simulink model "SAPF_pq_theory_Without_PI_Controller"  (R2023a)
settings: Solver=VariableStepAuto  StartTime=0.0  StopTime=2  RelTol=1e-3
libraries: spsThreePhaseVIMeasurementLib x3, spsSeriesRLCBranchLib x2, spsUniversalBridgeLib x2, dspfdesign x1, spsThreePhaseSeriesRLCBranchLib x1, spsThreePhaseSourceLib x1, spsVoltageMeasurementLib x1, sps_lib x1
settings Model: Creator=Nitiz Khanal  LastModifiedBy=Nitiz Khanal
settings DataIOCC: ReturnWorkspaceOutputs=off

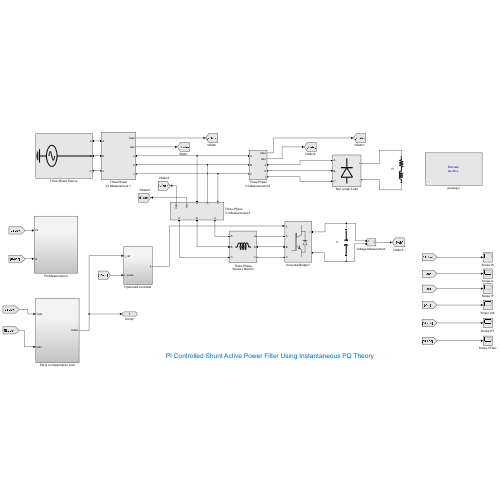
[thumbnail: Simulink's stored preview of the top-level diagram]
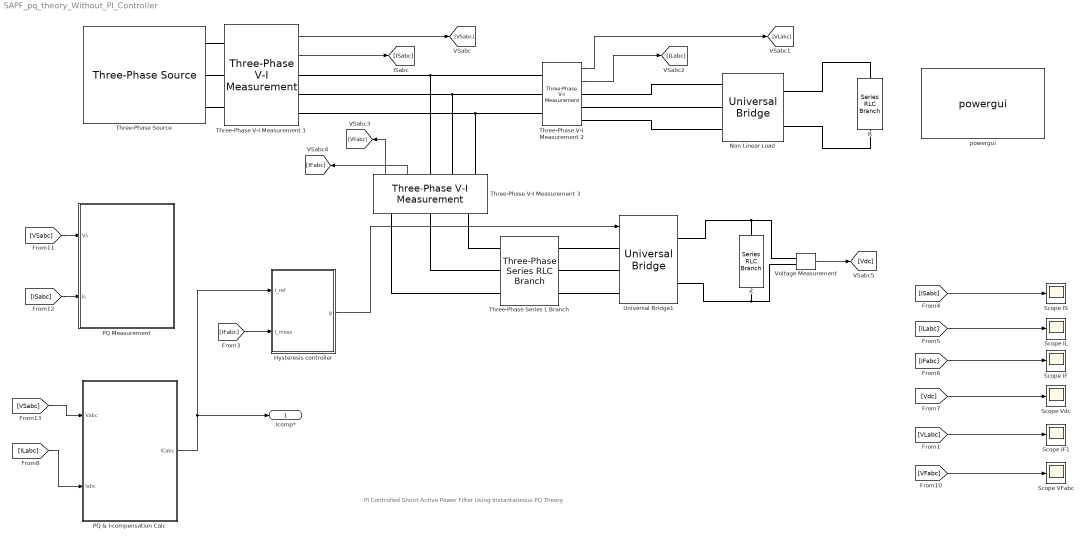
== system SAPF_pq_theory_Without_PI_Controller ==
  note: PI Controlled Shunt Active Power Filter Using Instantaneous PQ Theory
  C : spsSeriesRLCBranchLib/Series RLC Branch  LConnTagsString=__new0  RConnTagsString=__new0  BranchType=C  Resistance=1  Inductance=1e-3  SetiL0=off  InitialCurrent=0  Capacitance=1500e-6  Setx0=on  InitialVoltage=500  Measurements=None
  Hysteresis controller : Subsystem
  Non Linear Load : spsUniversalBridgeLib/Universal Bridge  Arms=3  SnubberResistance=1e5  SnubberCapacitance=inf  Device=Diodes  Ron=1e-3  Lon=0  ForwardVoltages="[  0  0  ]"  ForwardVoltage=0  GTOparameters=[ 10e-6 , 20e-6 ]  IGBTparameters=[ 1e-6 , 2e-6 ]  Measurements=None  Measurements_2=None  converterType=Rectifier
  PQ & I-compensation Calc : Subsystem
  PQ Measurement : Subsystem
  R : spsSeriesRLCBranchLib/Series RLC Branch  LConnTagsString=__new0  RConnTagsString=__new0  BranchType=RL  Resistance=30  Inductance=100e-3  SetiL0=off  InitialCurrent=0  Capacitance=1e-6  Setx0=off  InitialVoltage=0  Measurements=None
  Scope IF : Scope
  Scope IF1 : Scope
  Scope IL : Scope
  Scope IS : Scope
  Scope VFabc : Scope
  Scope Vdc : Scope
  Three-Phase Series L Branch : spsThreePhaseSeriesRLCBranchLib/Three-Phase Series RLC Branch  LConnTagsString=A|B|C  RConnTagsString=A|B|C  BranchType=L  Resistance=1  Inductance=2e-3  Capacitance=1e-6  Measurements=None
  "Three-Phase V-I Measurement 1 " : spsThreePhaseVIMeasurementLib/Three-Phase V-I Measurement  VoltageMeasurement=phase-to-ground  SetLabelV=off  LabelV=Vabc  Vpu=off  VpuLL=off  CurrentMeasurement=yes  SetLabelI=off  LabelI=Iabc  Ipu=off  Pbase=100e6  Vbase=500e3  OutputType=Complex  PhasorSimulation=off  PSBequivalent=0
  "Three-Phase V-I Measurement 2 " : spsThreePhaseVIMeasurementLib/Three-Phase V-I Measurement  VoltageMeasurement=phase-to-ground  SetLabelV=off  LabelV=Vabc  Vpu=off  VpuLL=off  CurrentMeasurement=yes  SetLabelI=off  LabelI=Iabc  Ipu=off  Pbase=100e6  Vbase=500e3  OutputType=Complex  PhasorSimulation=off  PSBequivalent=0
  Three-Phase V-I Measurement 3 : spsThreePhaseVIMeasurementLib/Three-Phase V-I Measurement  VoltageMeasurement=phase-to-ground  SetLabelV=off  LabelV=Vabc  Vpu=off  VpuLL=off  CurrentMeasurement=yes  SetLabelI=off  LabelI=Iabc  Ipu=off  Pbase=100e6  Vbase=500e3  OutputType=Complex  PhasorSimulation=off  PSBequivalent=0
  "Three-Phase Source " : spsThreePhaseSourceLib/Three-Phase Source  InternalConnection=Yg  VoltagePhases=off  Voltage=220  PhaseAngle=0  Voltage_phases=[25e3 25e3 25e3]/sqrt(3)  PhaseAngles_phases=[0 -120 +120]  Frequency=50  NonIdealSource=off  SpecifyImpedance=off  Resistance=0.8929  Inductance=16.58e-3  ShortCircuitLevel=100e6  BaseVoltage=25e3  XRratio=7  BusType=swing  Pref=10e3  Qref=0  Prefabc=[10e3, 10e3, 10e3]  Qrefabc=[0, 0, 0]  Qmin=-inf  Qmax=inf
  "Universal Bridge1 " : spsUniversalBridgeLib/Universal Bridge  Arms=3  SnubberResistance=1e5  SnubberCapacitance=inf  Device=IGBT / Diodes  Ron=1e-3  Lon=0  ForwardVoltages="[  0  0  ]"  ForwardVoltage=0  GTOparameters=[ 10e-6 , 20e-6 ]  IGBTparameters=[ 1e-6 , 2e-6 ]  Measurements=None  Measurements_2=None  converterType=Rectifier
  "Voltage Measurement " : spsVoltageMeasurementLib/Voltage Measurement  PhasorSimulation=off  OutputType=Complex  PSBequivalent=0
  powergui : sps_lib/powergui  Priority=1  SimulationMode=Discrete  SampleTime=2e-6  frequency=60  Iterations=50  frequencyindice=50  Pbase=100e6  ErrMax=1e-4  UnitsV=kV  UnitsW=MW  buscounter=0  FunctionMessages=off  echomessages=off  EnableUseOfTLC=off  CurrentSourceSwitches=off  DisableSnubberDevices=off  DisableRonSwitches=off  DisableVfSwitches=off  DisplayEquations=off  AutomaticDiscreteSolvers=off  SolverType=Tustin/Backward Euler (TBE)  Interpol=off  ExternalGateDelay=off  methode=off  Ts=100  x0status=blocks  SPID=on  SwTol=0  HookPort=off  NonlinearTolerance=1e-4  nMaxIteration=100  ContinueOnMaxIteration=off  RestoreLinks=warning  ResistiveCurrentMeasurement=off  Frange=[0:2:500]  Ylog=off  Xlog=on  ShowGrid=off  save=off  variable=ZData  structure=0  ZoomFFT=off  StartTime=0.0  cycles=1  DisplayStyle=1  fundamental=60  FreqAxis=off  MaxFrequency=1000  frequencyindicesteady=1  RmsSteady=1  display=off
  Icomp* : Outport
  wires:
  "Three-Phase V-I Measurement 1 "/1 -> [VSabc]
  "Three-Phase V-I Measurement 1 "/2 -> [ISabc]
  "Three-Phase V-I Measurement 2 "/1 -> [VLabc]
  "Three-Phase V-I Measurement 2 "/2 -> [ILabc]
  Three-Phase V-I Measurement 3/1 -> [VFabc]
  Three-Phase V-I Measurement 3/2 -> [IFabc]
  "Voltage Measurement "/1 -> [Vdc]
  Hysteresis controller/1(g) -> "Universal Bridge1 "/1
  [ISabc] -> Scope IS/1
  [ILabc] -> Scope IL/1
  [IFabc] -> Scope IF/1
  [Vdc] -> Scope Vdc/1
  [VSabc] -> PQ Measurement/1(Vs)
  [ISabc] -> PQ Measurement/2(Is)
  [VSabc] -> PQ & I-compensation Calc/1(Vabc)
  [IFabc] -> Hysteresis controller/2(I_meas)
  [ILabc] -> PQ & I-compensation Calc/2(Iabc)
  PQ & I-compensation Calc/1(ICabc) -> Hysteresis controller/1(I_ref), Icomp*/1
  [VLabc] -> Scope IF1/1
  [VFabc] -> Scope VFabc/1
  connections:
  "Three-Phase Source "/RConn1 -- "Three-Phase V-I Measurement 1 "/LConn1
  "Three-Phase Source "/RConn2 -- "Three-Phase V-I Measurement 1 "/LConn2
  "Three-Phase Source "/RConn3 -- "Three-Phase V-I Measurement 1 "/LConn3
  "Three-Phase V-I Measurement 1 "/RConn1 -- Three-Phase V-I Measurement 3/RConn1 -- "Three-Phase V-I Measurement 2 "/LConn1
  "Three-Phase V-I Measurement 1 "/RConn2 -- Three-Phase V-I Measurement 3/RConn2 -- "Three-Phase V-I Measurement 2 "/LConn2
  "Three-Phase V-I Measurement 1 "/RConn3 -- Three-Phase V-I Measurement 3/RConn3 -- "Three-Phase V-I Measurement 2 "/LConn3
  "Three-Phase V-I Measurement 2 "/RConn1 -- Non Linear Load/LConn1
  "Three-Phase V-I Measurement 2 "/RConn2 -- Non Linear Load/LConn2
  "Three-Phase V-I Measurement 2 "/RConn3 -- Non Linear Load/LConn3
  Non Linear Load/RConn1 -- R/LConn1
  Non Linear Load/RConn2 -- R/RConn1
  Three-Phase Series L Branch/RConn1 -- "Universal Bridge1 "/LConn1
  Three-Phase Series L Branch/RConn2 -- "Universal Bridge1 "/LConn2
  Three-Phase Series L Branch/RConn3 -- "Universal Bridge1 "/LConn3
  Three-Phase Series L Branch/LConn1 -- Three-Phase V-I Measurement 3/LConn3
  Three-Phase Series L Branch/LConn2 -- Three-Phase V-I Measurement 3/LConn2
  Three-Phase Series L Branch/LConn3 -- Three-Phase V-I Measurement 3/LConn1
  "Universal Bridge1 "/RConn1 -- "Voltage Measurement "/LConn1 -- C/LConn1
  "Universal Bridge1 "/RConn2 -- "Voltage Measurement "/LConn2 -- C/RConn1

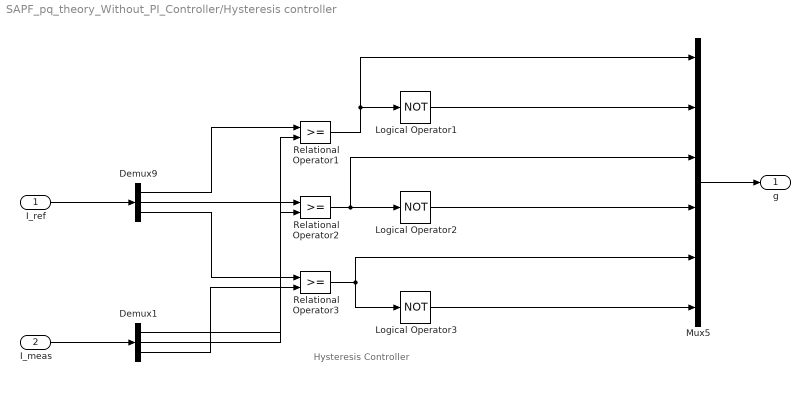
== system SAPF_pq_theory_Without_PI_Controller/Hysteresis controller ==
  note: Hysteresis Controller
  I_ref : Inport
  I_meas : Inport  Port=2
  Demux1 : Demux  Outputs=3
  Demux9 : Demux  Outputs=3
  Logical Operator1 : Logic  Operator=NOT  AllPortsSameDT=off  OutDataTypeStr=boolean
  Logical Operator2 : Logic  Operator=NOT  AllPortsSameDT=off  OutDataTypeStr=boolean
  Logical Operator3 : Logic  Operator=NOT  AllPortsSameDT=off  OutDataTypeStr=boolean
  Mux5 : Mux  Inputs=6
  Relational Operator1 : RelationalOperator  OutDataTypeStr=boolean  InputSameDT=off
  Relational Operator2 : RelationalOperator  OutDataTypeStr=boolean  InputSameDT=off
  Relational Operator3 : RelationalOperator  OutDataTypeStr=boolean  InputSameDT=off
  g : Outport
  wires:
  Relational Operator1/1 -> Logical Operator1/1, Mux5/1
  Relational Operator2/1 -> Logical Operator2/1, Mux5/3
  Relational Operator3/1 -> Logical Operator3/1, Mux5/5
  Demux9/1 -> Relational Operator1/1
  Demux9/3 -> Relational Operator3/1
  Logical Operator1/1 -> Mux5/2
  Logical Operator2/1 -> Mux5/4
  Logical Operator3/1 -> Mux5/6
  Mux5/1 -> g/1
  Demux9/2 -> Relational Operator2/1
  Demux1/1 -> Relational Operator1/2
  Demux1/2 -> Relational Operator2/2
  Demux1/3 -> Relational Operator3/2
  I_ref/1 -> Demux9/1
  I_meas/1 -> Demux1/1

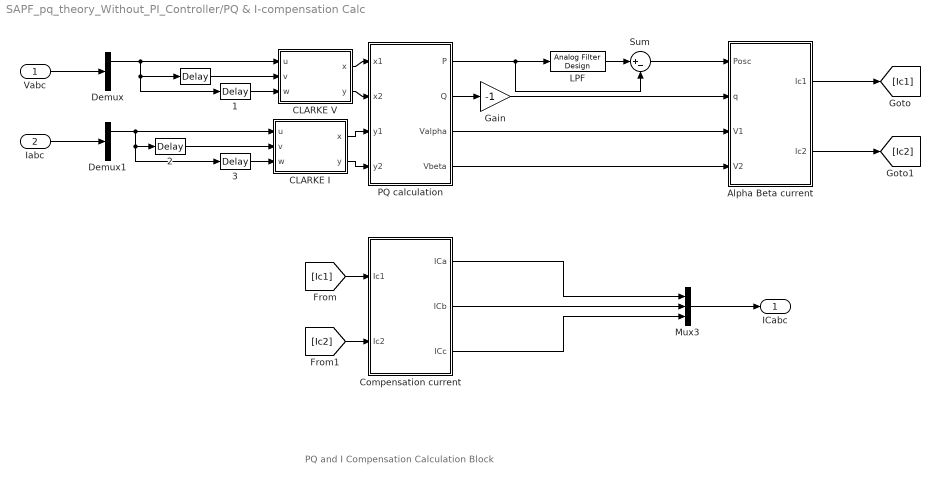
== system SAPF_pq_theory_Without_PI_Controller/PQ & I-compensation Calc ==
  note: PQ and I Compensation Calculation Block
  Vabc : Inport
  Iabc : Inport  Port=2
  " " : TransportDelay  DelayTime=0.006666666  BufferSize=4096
  " 1" : TransportDelay  DelayTime=0.013333333  BufferSize=7168
  " 2" : TransportDelay  DelayTime=0.006666666  BufferSize=4096
  " 3" : TransportDelay  DelayTime=0.013333333
  Alpha Beta current : MATLAB Function  TreatAsAtomicUnit=on
  CLARKE I : MATLAB Function  TreatAsAtomicUnit=on
  CLARKE V : MATLAB Function  TreatAsAtomicUnit=on
  Compensation current : MATLAB Function  TreatAsAtomicUnit=on
  Demux : Demux  Outputs=3
  Demux1 : Demux  Outputs=3
  Gain : Gain  Gain=-1
  LPF : dspfdesign/Analog Filter Design  method=Butterworth  filttype=Lowpass  N=5  Wlo=2*pi*50  Whi=80  Rp=2  Rs=40
  Mux3 : Mux  Inputs=3
  PQ calculation : MATLAB Function  TreatAsAtomicUnit=on
  Sum : Sum  Inputs=|+-
  ICabc : Outport
  wires:
  Iabc/1 -> Demux1/1
  Vabc/1 -> Demux/1
  [Ic1] -> Compensation current/1(Ic1)
  [Ic2] -> Compensation current/2(Ic2)
  Compensation current/1(ICa) -> Mux3/1
  Compensation current/2(ICb) -> Mux3/2
  Compensation current/3(ICc) -> Mux3/3
  CLARKE V/1(x) -> PQ calculation/1(x1)
  CLARKE V/2(y) -> PQ calculation/2(x2)
  CLARKE I/1(x) -> PQ calculation/3(y1)
  PQ calculation/2(Q) -> Gain/1
  PQ calculation/1(P) -> Sum/2, LPF/1
  Gain/1 -> Alpha Beta current/2(q)
  PQ calculation/3(Valpha) -> Alpha Beta current/3(V1)
  Alpha Beta current/1(Ic1) -> [Ic1]
  Alpha Beta current/2(Ic2) -> [Ic2]
  CLARKE I/2(y) -> PQ calculation/4(y2)
  PQ calculation/4(Vbeta) -> Alpha Beta current/4(V2)
  Demux/1 -> CLARKE V/1(u), " 1"/1, " "/1
  Demux1/1 -> CLARKE I/1(u), " 3"/1, " 2"/1
  Sum/1 -> Alpha Beta current/1(Posc)
  Mux3/1 -> ICabc/1
  " "/1 -> CLARKE V/2(v)
  " 1"/1 -> CLARKE V/3(w)
  " 2"/1 -> CLARKE I/2(v)
  " 3"/1 -> CLARKE I/3(w)
  LPF/1 -> Sum/1

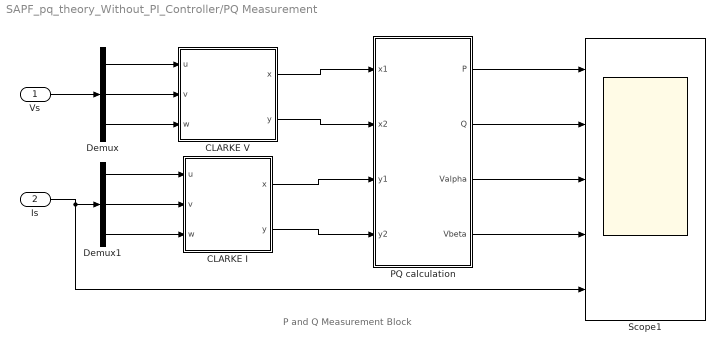
== system SAPF_pq_theory_Without_PI_Controller/PQ Measurement ==
  note: P and Q Measurement Block
  Vs : Inport
  Is : Inport  Port=2
  CLARKE I : MATLAB Function  TreatAsAtomicUnit=on
  CLARKE V : MATLAB Function  TreatAsAtomicUnit=on
  Demux : Demux  Outputs=3
  Demux1 : Demux  Outputs=3
  PQ calculation : MATLAB Function  TreatAsAtomicUnit=on
  "Scope1 " : Scope  NumInputPorts=5
  wires:
  CLARKE V/1(x) -> PQ calculation/1(x1)
  CLARKE V/2(y) -> PQ calculation/2(x2)
  CLARKE I/1(x) -> PQ calculation/3(y1)
  CLARKE I/2(y) -> PQ calculation/4(y2)
  Demux/1 -> CLARKE V/1(u)
  Demux/2 -> CLARKE V/2(v)
  Demux/3 -> CLARKE V/3(w)
  Demux1/1 -> CLARKE I/1(u)
  Demux1/2 -> CLARKE I/2(v)
  Demux1/3 -> CLARKE I/3(w)
  Vs/1 -> Demux/1
  Is/1 -> Demux1/1, "Scope1 "/5
  PQ calculation/1(P) -> "Scope1 "/1
  PQ calculation/2(Q) -> "Scope1 "/2
  PQ calculation/3(Valpha) -> "Scope1 "/3
  PQ calculation/4(Vbeta) -> "Scope1 "/4

== matlab function SAPF_pq_theory_Without_PI_Controller/PQ Measurement/CLARKE I ==
  data: u input; x output; v input; w input; y output
function [x,y] = ICT(u,v,w)
%#em1

x = sqrt(2/3)*(u-(0.5*v)-(0.5*w));
y = sqrt(2)*(0+(0.5*v)-(0.5*w));

== matlab function SAPF_pq_theory_Without_PI_Controller/PQ Measurement/CLARKE V ==
  data: u input; x output; v input; w input; y output
function [x,y] = VCT(u,v,w)
%#em1

x = sqrt(2/3)*(u-(0.5*v)-(0.5*w));
y = sqrt(2)*(0+(0.5*v)-(0.5*w));

== matlab function SAPF_pq_theory_Without_PI_Controller/PQ Measurement/PQ calculation ==
  data: x1 input; P output; Q output; x2 input; y1 input; y2 input; Valpha output; Vbeta output
function [P,Q,Valpha,Vbeta] = PQ(x1,x2,y1,y2)
%#em1

P = (x1*y1)+(x2*y2);
Q = (x2*y1)-(x1*y2);
Valpha = x1;
Vbeta = x2;

== matlab function SAPF_pq_theory_Without_PI_Controller/PQ & I-compensation Calc/Alpha Beta current ==
  data: Posc input; Ic1 output; q input; V1 input; Ic2 output; V2 input
function [Ic1, Ic2] = ICOM(Posc, q, V1, V2)
    % Posc is the oscillating component of active power (p_tilde)
    % q is the instantaneous reactive power
    % V1 and V2 are alpha and beta components of voltage
    
    denominator = V1^2 + V2^2;
    
    % Calculate compensation currents directly using oscillating power components
    Ic1 = (V1 * Posc + V2 * q) / denominator;
    Ic2 = (V2 * Posc - V1 * q) / denominator;
end

== matlab function SAPF_pq_theory_Without_PI_Controller/PQ & I-compensation Calc/CLARKE I ==
  data: u input; x output; v input; w input; y output
function [x,y] = ICT(u,v,w)
%#em1

x = sqrt(2/3)*(u-(0.5*v)-(0.5*w));
y = sqrt(2)*(0+(0.5*v)-(0.5*w));

== matlab function SAPF_pq_theory_Without_PI_Controller/PQ & I-compensation Calc/CLARKE V ==
  data: u input; x output; v input; w input; y output
function [x,y] = VCT(u,v,w)
%#em1

x = sqrt(2/3)*(u-(0.5*v)-(0.5*w));
y = sqrt(2)*(0+(0.5*v)-(0.5*w));

== matlab function SAPF_pq_theory_Without_PI_Controller/PQ & I-compensation Calc/Compensation current ==
  data: Ic1 input; ICa output; Ic2 input; ICb output; ICc output
function [ICa,ICb,ICc] = Ical(Ic1,Ic2)
%#em1

ICa = sqrt(2/3)*(Ic1);
ICb = sqrt(2/3)*((-0.5*Ic1)+((sqrt(3)/2)*Ic2));
ICc = sqrt(2/3)*((-0.5*Ic1)-((sqrt(3)/2)*Ic2));

== matlab function SAPF_pq_theory_Without_PI_Controller/PQ & I-compensation Calc/PQ calculation ==
  data: x1 input; P output; Q output; x2 input; y1 input; y2 input; Valpha output; Vbeta output
function [P,Q,Valpha,Vbeta] = PQ(x1,x2,y1,y2)
%#em1

P = (x1*y1)+(x2*y2);
Q = (x2*y1)-(x1*y2);
Valpha = x1;
Vbeta = x2;
